simulink model "FOC"  (R2024b)
settings: Solver=ode4  StartTime=0.0  StopTime=0.5  FixedStep=Ts/10  RelTol=1e-3
InitFcn:
  | foc_param;
undefined symbols (not defined in the file): DiscIntNeverNeededParam, Iq_max, Ki_dq, Ki_w, Kp_dq, Kp_w, Spd_ref_tau, Ts, Vmax
settings Model: Creator=BitCore  LastModifiedBy=BitCore

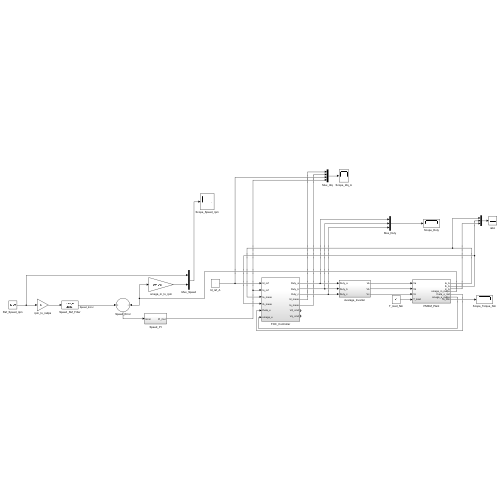
[thumbnail: Simulink's stored preview of the top-level diagram]
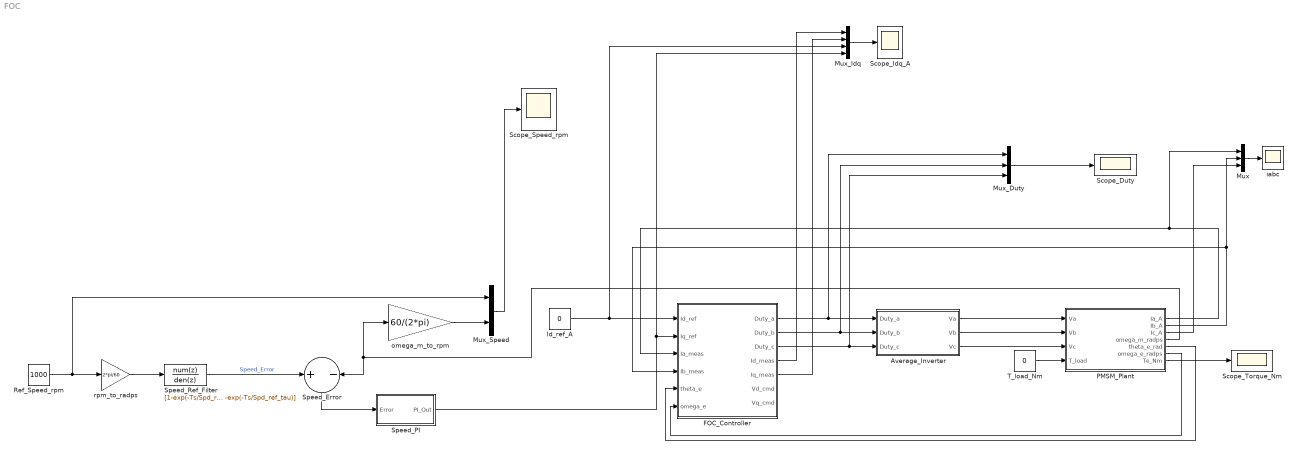
== system FOC ==
  Average_Inverter : Subsystem
  FOC_Controller : Subsystem
  Id_ref_A : Constant  Value=0
  Mux : Mux  Inputs=3
  Mux_Duty : Mux  Inputs=3
  Mux_Idq : Mux
  Mux_Speed : Mux  Inputs=2
  PMSM_Plant : Subsystem
  Ref_Speed_rpm : Constant  Value=1000
  Scope_Duty : Scope
  Scope_Idq_A : Scope
  Scope_Speed_rpm : Scope
  Scope_Torque_Nm : Scope
  Speed_Error : Sum  Inputs=+-
  Speed_PI : Subsystem
  Speed_Ref_Filter : DiscreteTransferFcn  Numerator=[1-exp(-Ts/Spd_ref_tau)]  Denominator=[1 -exp(-Ts/Spd_ref_tau)]  SampleTime=Ts
  T_load_Nm : Constant  Value=0
  iabc : Scope
  omega_m_to_rpm : Gain  Gain=60/(2*pi)
  rpm_to_radps : Gain  Gain=2*pi/60
  wires:
  Speed_Ref_Filter/1 -> Speed_Error/1  "Speed_Error"
  Mux/1 -> iabc/1
  Mux_Duty/1 -> Scope_Duty/1
  Average_Inverter/3(Vc) -> PMSM_Plant/3(Vc)
  FOC_Controller/1(Duty_a) -> Mux_Duty/1, Average_Inverter/1(Duty_a)
  Mux_Idq/1 -> Scope_Idq_A/1
  FOC_Controller/2(Duty_b) -> Mux_Duty/2, Average_Inverter/2(Duty_b)
  FOC_Controller/4(Id_meas) -> Mux_Idq/1
  Speed_PI/1(PI_Out) -> Mux_Idq/4, FOC_Controller/2(Iq_ref)
  Id_ref_A/1 -> Mux_Idq/3, FOC_Controller/1(Id_ref)
  Speed_Error/1 -> Speed_PI/1(Error)
  Average_Inverter/1(Va) -> PMSM_Plant/1(Va)
  PMSM_Plant/1(Ia_A) -> Mux/1, FOC_Controller/3(Ia_meas)
  Average_Inverter/2(Vb) -> PMSM_Plant/2(Vb)
  PMSM_Plant/4(omega_m_radps) -> omega_m_to_rpm/1, Speed_Error/2
  T_load_Nm/1 -> PMSM_Plant/4(T_load)
  PMSM_Plant/6(omega_e_radps) -> FOC_Controller/6(omega_e)
  PMSM_Plant/7(Te_Nm) -> Scope_Torque_Nm/1
  PMSM_Plant/5(theta_e_rad) -> FOC_Controller/5(theta_e)
  FOC_Controller/3(Duty_c) -> Mux_Duty/3, Average_Inverter/3(Duty_c)
  FOC_Controller/5(Iq_meas) -> Mux_Idq/2
  Mux_Speed/1 -> Scope_Speed_rpm/1
  PMSM_Plant/3(Ic_A) -> Mux/3
  rpm_to_radps/1 -> Speed_Ref_Filter/1
  Ref_Speed_rpm/1 -> Mux_Speed/1, rpm_to_radps/1
  PMSM_Plant/2(Ib_A) -> Mux/2, FOC_Controller/4(Ib_meas)
  omega_m_to_rpm/1 -> Mux_Speed/2

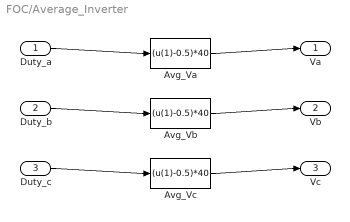
== system FOC/Average_Inverter ==
  Duty_a : Inport
  Duty_b : Inport  Port=2
  Duty_c : Inport  Port=3
  Avg_Va : Fcn  Expr=(u(1)-0.5)*40
  Avg_Vb : Fcn  Expr=(u(1)-0.5)*40
  Avg_Vc : Fcn  Expr=(u(1)-0.5)*40
  Va : Outport
  Vb : Outport  Port=2
  Vc : Outport  Port=3
  wires:
  Duty_a/1 -> Avg_Va/1
  Avg_Va/1 -> Va/1
  Duty_b/1 -> Avg_Vb/1
  Avg_Vb/1 -> Vb/1
  Duty_c/1 -> Avg_Vc/1
  Avg_Vc/1 -> Vc/1

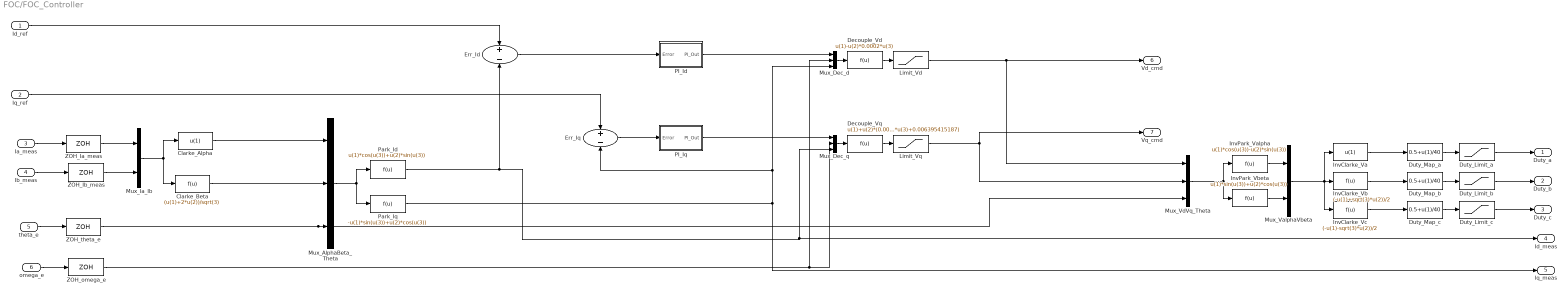
== system FOC/FOC_Controller ==
  Id_ref : Inport
  Iq_ref : Inport  Port=2
  Ia_meas : Inport  Port=3
  Ib_meas : Inport  Port=4
  theta_e : Inport  Port=5
  omega_e : Inport  Port=6
  Clarke_Alpha : Fcn  Expr=u(1)
  Clarke_Beta : Fcn  Expr=(u(1)+2*u(2))/sqrt(3)
  Decouple_Vd : Fcn  Expr=u(1)-u(2)*0.0002*u(3)
  Decouple_Vq : Fcn  Expr=u(1)+u(2)*(0.0002*u(3)+0.006395415187)
  Duty_Limit_a : Saturate  UpperLimit=1  LowerLimit=0
  Duty_Limit_b : Saturate  UpperLimit=1  LowerLimit=0
  Duty_Limit_c : Saturate  UpperLimit=1  LowerLimit=0
  Duty_Map_a : Fcn  Expr=0.5+u(1)/40
  Duty_Map_b : Fcn  Expr=0.5+u(1)/40
  Duty_Map_c : Fcn  Expr=0.5+u(1)/40
  Err_Id : Sum  Inputs=+-
  Err_Iq : Sum  Inputs=+-
  InvClarke_Va : Fcn  Expr=u(1)
  InvClarke_Vb : Fcn  Expr=(-u(1)+sqrt(3)*u(2))/2
  InvClarke_Vc : Fcn  Expr=(-u(1)-sqrt(3)*u(2))/2
  InvPark_Valpha : Fcn  Expr=u(1)*cos(u(3))-u(2)*sin(u(3))
  InvPark_Vbeta : Fcn  Expr=u(1)*sin(u(3))+u(2)*cos(u(3))
  Limit_Vd : Saturate  UpperLimit=Vmax  LowerLimit=-Vmax
  Limit_Vq : Saturate  UpperLimit=Vmax  LowerLimit=-Vmax
  Mux_AlphaBeta_Theta : Mux  Inputs=3
  Mux_Dec_d : Mux  Inputs=3
  Mux_Dec_q : Mux  Inputs=3
  Mux_Ia_Ib : Mux  Inputs=2
  Mux_ValphaVbeta : Mux  Inputs=2
  Mux_VdVq_Theta : Mux  Inputs=3
  PI_Id : Subsystem
  PI_Iq : Subsystem
  Park_Id : Fcn  Expr=u(1)*cos(u(3))+u(2)*sin(u(3))
  Park_Iq : Fcn  Expr=-u(1)*sin(u(3))+u(2)*cos(u(3))
  ZOH_Ia_meas : ZeroOrderHold  SampleTime=Ts
  ZOH_Ib_meas : ZeroOrderHold  SampleTime=Ts
  ZOH_omega_e : ZeroOrderHold  SampleTime=Ts
  ZOH_theta_e : ZeroOrderHold  SampleTime=Ts
  Duty_a : Outport
  Duty_b : Outport  Port=2
  Duty_c : Outport  Port=3
  Id_meas : Outport  Port=4
  Iq_meas : Outport  Port=5
  Vd_cmd : Outport  Port=6
  Vq_cmd : Outport  Port=7
  wires:
  Ia_meas/1 -> ZOH_Ia_meas/1
  Ib_meas/1 -> ZOH_Ib_meas/1
  theta_e/1 -> ZOH_theta_e/1
  omega_e/1 -> ZOH_omega_e/1
  ZOH_Ia_meas/1 -> Mux_Ia_Ib/1
  ZOH_Ib_meas/1 -> Mux_Ia_Ib/2
  Mux_Ia_Ib/1 -> Clarke_Alpha/1, Clarke_Beta/1
  Clarke_Alpha/1 -> Mux_AlphaBeta_Theta/1
  Clarke_Beta/1 -> Mux_AlphaBeta_Theta/2
  ZOH_theta_e/1 -> Mux_VdVq_Theta/3, Mux_AlphaBeta_Theta/3
  Mux_AlphaBeta_Theta/1 -> Park_Id/1, Park_Iq/1
  Id_ref/1 -> Err_Id/1
  Park_Id/1 -> Id_meas/1, Mux_Dec_q/3, Err_Id/2
  Iq_ref/1 -> Err_Iq/1
  Park_Iq/1 -> Iq_meas/1, Mux_Dec_d/3, Err_Iq/2
  Err_Id/1 -> PI_Id/1(Error)
  Err_Iq/1 -> PI_Iq/1(Error)
  PI_Id/1(PI_Out) -> Mux_Dec_d/1
  ZOH_omega_e/1 -> Mux_Dec_d/2, Mux_Dec_q/2
  PI_Iq/1(PI_Out) -> Mux_Dec_q/1
  Mux_Dec_d/1 -> Decouple_Vd/1
  Mux_Dec_q/1 -> Decouple_Vq/1
  Decouple_Vd/1 -> Limit_Vd/1
  Decouple_Vq/1 -> Limit_Vq/1
  Limit_Vd/1 -> Vd_cmd/1, Mux_VdVq_Theta/1
  Limit_Vq/1 -> Vq_cmd/1, Mux_VdVq_Theta/2
  Mux_VdVq_Theta/1 -> InvPark_Vbeta/1, InvPark_Valpha/1
  InvPark_Valpha/1 -> Mux_ValphaVbeta/1
  InvPark_Vbeta/1 -> Mux_ValphaVbeta/2
  Mux_ValphaVbeta/1 -> InvClarke_Vc/1, InvClarke_Va/1, InvClarke_Vb/1
  InvClarke_Va/1 -> Duty_Map_a/1
  Duty_Map_a/1 -> Duty_Limit_a/1
  Duty_Limit_a/1 -> Duty_a/1
  InvClarke_Vb/1 -> Duty_Map_b/1
  Duty_Map_b/1 -> Duty_Limit_b/1
  Duty_Limit_b/1 -> Duty_b/1
  InvClarke_Vc/1 -> Duty_Map_c/1
  Duty_Map_c/1 -> Duty_Limit_c/1
  Duty_Limit_c/1 -> Duty_c/1

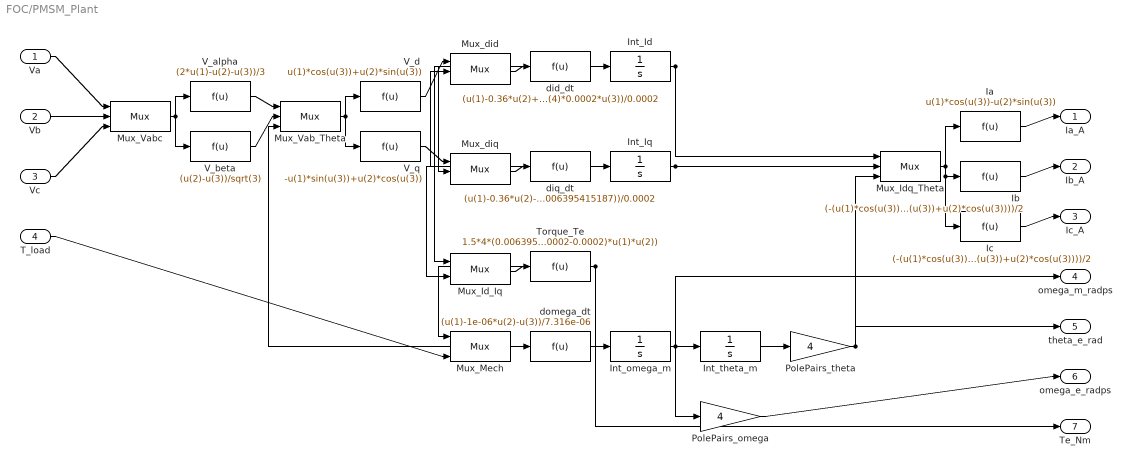
== system FOC/PMSM_Plant ==
  Va : Inport
  Vb : Inport  Port=2
  Vc : Inport  Port=3
  T_load : Inport  Port=4
  Ia : Fcn  Expr=u(1)*cos(u(3))-u(2)*sin(u(3))
  Ib : Fcn  Expr=(-(u(1)*cos(u(3))-u(2)*sin(u(3)))+sqrt(3)*(u(1)*sin(u(3))+u(2)*cos(u(3))))/2
  Ic : Fcn  Expr=(-(u(1)*cos(u(3))-u(2)*sin(u(3)))-sqrt(3)*(u(1)*sin(u(3))+u(2)*cos(u(3))))/2
  Int_Id : Integrator
  Int_Iq : Integrator
  Int_omega_m : Integrator
  Int_theta_m : Integrator
  Mux_Id_Iq : Mux  Inputs=2
  Mux_Idq_Theta : Mux  Inputs=3
  Mux_Mech : Mux  Inputs=3
  Mux_Vab_Theta : Mux  Inputs=3
  Mux_Vabc : Mux  Inputs=3
  Mux_did : Mux
  Mux_diq : Mux
  PolePairs_omega : Gain  Gain=4
  PolePairs_theta : Gain  Gain=4
  Torque_Te : Fcn  Expr=1.5*4*(0.006395415187*u(2)+(0.0002-0.0002)*u(1)*u(2))
  V_alpha : Fcn  Expr=(2*u(1)-u(2)-u(3))/3
  V_beta : Fcn  Expr=(u(2)-u(3))/sqrt(3)
  V_d : Fcn  Expr=u(1)*cos(u(3))+u(2)*sin(u(3))
  V_q : Fcn  Expr=-u(1)*sin(u(3))+u(2)*cos(u(3))
  did_dt : Fcn  Expr=(u(1)-0.36*u(2)+u(4)*0.0002*u(3))/0.0002
  diq_dt : Fcn  Expr=(u(1)-0.36*u(2)-u(4)*(0.0002*u(3)+0.006395415187))/0.0002
  domega_dt : Fcn  Expr=(u(1)-1e-06*u(2)-u(3))/7.316e-06
  Ia_A : Outport
  Ib_A : Outport  Port=2
  Ic_A : Outport  Port=3
  omega_m_radps : Outport  Port=4
  theta_e_rad : Outport  Port=5
  omega_e_radps : Outport  Port=6
  Te_Nm : Outport  Port=7
  wires:
  Va/1 -> Mux_Vabc/1
  Vb/1 -> Mux_Vabc/2
  Vc/1 -> Mux_Vabc/3
  Mux_Vabc/1 -> V_alpha/1, V_beta/1
  V_alpha/1 -> Mux_Vab_Theta/1
  V_beta/1 -> Mux_Vab_Theta/2
  Mux_Vab_Theta/1 -> V_d/1, V_q/1
  V_d/1 -> Mux_did/1
  Int_Id/1 -> Mux_did/2, Mux_diq/3, Mux_Id_Iq/1, Mux_Idq_Theta/1
  Int_Iq/1 -> Mux_did/3, Mux_diq/2, Mux_Id_Iq/2, Mux_Idq_Theta/2
  V_q/1 -> Mux_diq/1
  Mux_did/1 -> did_dt/1
  did_dt/1 -> Int_Id/1
  Mux_diq/1 -> diq_dt/1
  diq_dt/1 -> Int_Iq/1
  Mux_Id_Iq/1 -> Torque_Te/1
  Torque_Te/1 -> Mux_Mech/1, Te_Nm/1
  Int_omega_m/1 -> Mux_Mech/2, Int_theta_m/1, PolePairs_omega/1, omega_m_radps/1
  T_load/1 -> Mux_Mech/3
  Mux_Mech/1 -> domega_dt/1
  domega_dt/1 -> Int_omega_m/1
  Int_theta_m/1 -> PolePairs_theta/1
  PolePairs_theta/1 -> Mux_Vab_Theta/3, Mux_Idq_Theta/3, theta_e_rad/1
  Mux_Idq_Theta/1 -> Ib/1, Ic/1, Ia/1
  Ia/1 -> Ia_A/1
  Ib/1 -> Ib_A/1
  Ic/1 -> Ic_A/1
  PolePairs_omega/1 -> omega_e_radps/1

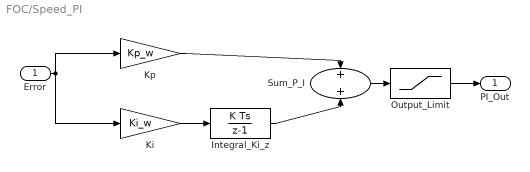
== system FOC/Speed_PI ==
  Error : Inport
  Integral_Ki_z : DiscreteIntegrator  SampleTime=Ts  LimitOutput=on  UpperSaturationLimit=Iq_max  LowerSaturationLimit=-Iq_max  ICPrevOutput=DiscIntNeverNeededParam  ICPrevScaledInput=DiscIntNeverNeededParam
  Ki : Gain  Gain=Ki_w
  Kp : Gain  Gain=Kp_w
  Output_Limit : Saturate  UpperLimit=Iq_max  LowerLimit=-Iq_max
  Sum_P_I : Sum
  PI_Out : Outport
  wires:
  Error/1 -> Kp/1, Ki/1
  Ki/1 -> Integral_Ki_z/1
  Kp/1 -> Sum_P_I/1
  Integral_Ki_z/1 -> Sum_P_I/2
  Sum_P_I/1 -> Output_Limit/1
  Output_Limit/1 -> PI_Out/1

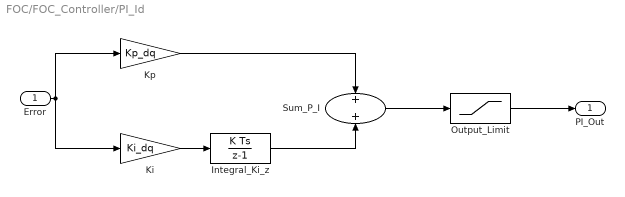
== system FOC/FOC_Controller/PI_Id ==
  Error : Inport
  Integral_Ki_z : DiscreteIntegrator  SampleTime=Ts  LimitOutput=on  UpperSaturationLimit=Vmax  LowerSaturationLimit=-Vmax  ICPrevOutput=DiscIntNeverNeededParam  ICPrevScaledInput=DiscIntNeverNeededParam
  Ki : Gain  Gain=Ki_dq
  Kp : Gain  Gain=Kp_dq
  Output_Limit : Saturate  UpperLimit=Vmax  LowerLimit=-Vmax
  Sum_P_I : Sum
  PI_Out : Outport
  wires:
  Error/1 -> Kp/1, Ki/1
  Ki/1 -> Integral_Ki_z/1
  Kp/1 -> Sum_P_I/1
  Integral_Ki_z/1 -> Sum_P_I/2
  Sum_P_I/1 -> Output_Limit/1
  Output_Limit/1 -> PI_Out/1

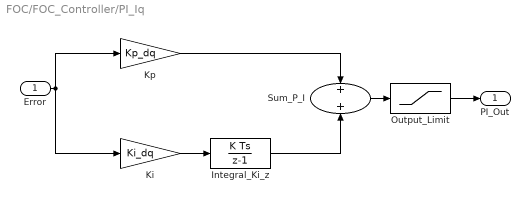
== system FOC/FOC_Controller/PI_Iq ==
  Error : Inport
  Integral_Ki_z : DiscreteIntegrator  SampleTime=Ts  LimitOutput=on  UpperSaturationLimit=Vmax  LowerSaturationLimit=-Vmax  ICPrevOutput=DiscIntNeverNeededParam  ICPrevScaledInput=DiscIntNeverNeededParam
  Ki : Gain  Gain=Ki_dq
  Kp : Gain  Gain=Kp_dq
  Output_Limit : Saturate  UpperLimit=Vmax  LowerLimit=-Vmax
  Sum_P_I : Sum
  PI_Out : Outport
  wires:
  Error/1 -> Kp/1, Ki/1
  Ki/1 -> Integral_Ki_z/1
  Kp/1 -> Sum_P_I/1
  Integral_Ki_z/1 -> Sum_P_I/2
  Sum_P_I/1 -> Output_Limit/1
  Output_Limit/1 -> PI_Out/1
